simulink model "mppt"  (R2022b)
settings: Solver=ode23tb  StartTime=0.0  StopTime=0.5  RelTol=1e-3
libraries: spsSeriesRLCBranchLib x7, spsCurrentMeasurementLib x4, spsVoltageMeasurementLib x4, spsDiodeLib x2, spsIGBTDiodeLib x2, simulink x2, spsFuelCellStackLib x1, spsDCVoltageSourceLib x1, spspowerguiLib x1
settings Model: Creator=gobis  LastModifiedBy=gobis
settings SolverCC: ZeroCrossAlgorithm=Adaptive
settings DebuggingCC: MaskedZcDiagnostic=none  IgnoredZcDiagnostic=none

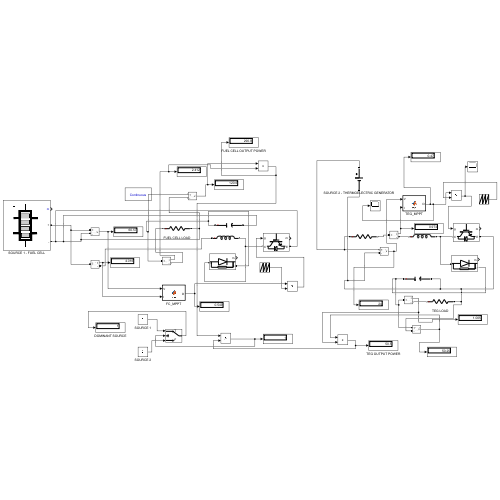
[thumbnail: Simulink's stored preview of the top-level diagram]
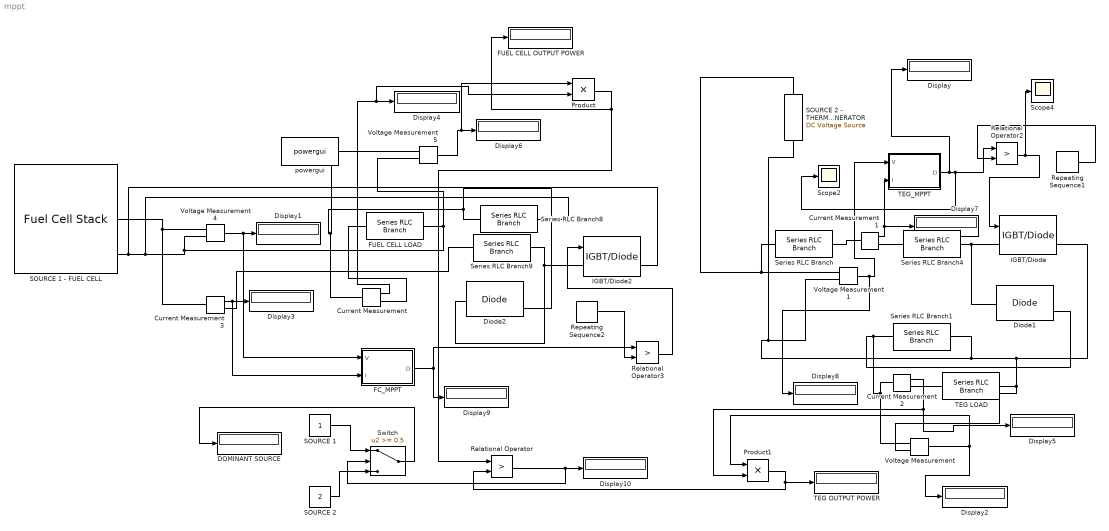
== system mppt ==
  Current Measurement{,1..3} (4 alike) : spsCurrentMeasurementLib/Current Measurement  PhasorSimulation=off  OutputType=Complex  PSBequivalent=0
  DOMINANT SOURCE : Display
  Diode1 : spsDiodeLib/Diode  Ron=0.001  Lon=0  Vf=0.8  IC=0  UseSnubber=0  Rs=500  Cs=250e-9  Measurements=on
  Diode2 : spsDiodeLib/Diode  Ron=0.001  Lon=0  Vf=0.8  IC=0  UseSnubber=0  Rs=500  Cs=250e-9  Measurements=on
  Display{,1..10} (11 alike) : Display
  FC_MPPT : MATLAB Function  TreatAsAtomicUnit=on
  FUEL CELL LOAD : spsSeriesRLCBranchLib/Series RLC Branch  LConnTagsString=__new0  RConnTagsString=__new0  BranchType=R  Resistance=50  Inductance=1e-3  SetiL0=off  InitialCurrent=0  Capacitance=1e-6  Setx0=off  InitialVoltage=0  Measurements=None
  FUEL CELL OUTPUT POWER : Display
  IGBT/Diode : spsIGBTDiodeLib/IGBT//Diode  Ron=1e-3  Rs=1e5  Cs=inf  Measurements=on
  IGBT/Diode2 : spsIGBTDiodeLib/IGBT//Diode  Ron=1e-3  Rs=1e5  Cs=inf  Measurements=on
  Product : Product
  Product1 : Product
  Relational Operator : RelationalOperator  Operator=>  OutDataTypeStr=boolean  RndMeth=Simplest  InputSameDT=off
  Relational Operator2 : RelationalOperator  Operator=>  OutDataTypeStr=boolean  RndMeth=Simplest  InputSameDT=off
  Relational Operator3 : RelationalOperator  Operator=>  OutDataTypeStr=boolean  RndMeth=Simplest  InputSameDT=off
  Repeating Sequence1 : simulink/Sources/Repeating Sequence  rep_seq_t=[0 0.0001]  rep_seq_y=[0 1]
  Repeating Sequence2 : simulink/Sources/Repeating Sequence  rep_seq_t=[0 0.0001]  rep_seq_y=[0 1]
  SOURCE 1 : Constant
  SOURCE 1 - FUEL CELL : spsFuelCellStackLib/Fuel Cell Stack  PresetModel=No (User-Defined)  FcType=0  Detailed=Detailed  Eoc=[65,63]  NomVI=[133.3,45]  EndVI=[225,37]  Nc=65  n=55  TOp=65  AirFr=300  SuppPress=[1.5,1]  Comp=[99.95,21,1]  SignX=off  SignY=off  FlowRateH2=off  FlowRateAir=off  SystemTemp=off  SystemPH2=off  SystemPAir=off  FCDyn=off  FC_tau=1  Peak_O2=80  V_Under=10
      settings: LibrarySourceBlock=sps_lib/Sources/Fuel Cell Stack
  SOURCE 2 : Constant  Value=2
  SOURCE 2 - THERMOELECTRIC GENERATOR : spsDCVoltageSourceLib/DC Voltage Source  Amplitude=24  Measurements=None
  Scope2 : Scope
  Scope4 : Scope
  Series RLC Branch : spsSeriesRLCBranchLib/Series RLC Branch  LConnTagsString=__new0  RConnTagsString=__new0  BranchType=R  Resistance=1  Inductance=1e-3  SetiL0=off  InitialCurrent=0  Capacitance=1e-6  Setx0=off  InitialVoltage=0  Measurements=None
  Series RLC Branch1 : spsSeriesRLCBranchLib/Series RLC Branch  LConnTagsString=__new0  RConnTagsString=__new0  BranchType=C  Resistance=1  Inductance=1e-3  SetiL0=off  InitialCurrent=0  Capacitance=1e-6  Setx0=off  InitialVoltage=0  Measurements=None
  Series RLC Branch4 : spsSeriesRLCBranchLib/Series RLC Branch  LConnTagsString=__new0  RConnTagsString=__new0  BranchType=L  Resistance=1  Inductance=1e-3  SetiL0=off  InitialCurrent=0  Capacitance=1e-6  Setx0=off  InitialVoltage=0  Measurements=None
  Series RLC Branch8 : spsSeriesRLCBranchLib/Series RLC Branch  LConnTagsString=__new0  RConnTagsString=__new0  BranchType=C  Resistance=1  Inductance=1e-3  SetiL0=off  InitialCurrent=0  Capacitance=470e-6  Setx0=off  InitialVoltage=0  Measurements=None
  Series RLC Branch9 : spsSeriesRLCBranchLib/Series RLC Branch  LConnTagsString=__new0  RConnTagsString=__new0  BranchType=L  Resistance=1  Inductance=1e-3  SetiL0=off  InitialCurrent=0  Capacitance=1e-6  Setx0=off  InitialVoltage=0  Measurements=None
  Switch : Switch  Threshold=0.5  SaturateOnIntegerOverflow=off  InputSameDT=off
  TEG LOAD : spsSeriesRLCBranchLib/Series RLC Branch  LConnTagsString=__new0  RConnTagsString=__new0  BranchType=R  Resistance=50  Inductance=1e-3  SetiL0=off  InitialCurrent=0  Capacitance=1e-6  Setx0=off  InitialVoltage=0  Measurements=None
  TEG OUTPUT POWER : Display
  TEG_MPPT : MATLAB Function  TreatAsAtomicUnit=on
  Voltage Measurement{,1,4..5} (4 alike) : spsVoltageMeasurementLib/Voltage Measurement  PhasorSimulation=off  OutputType=Complex  PSBequivalent=0
  powergui : spspowerguiLib/powergui  Priority=1  SimulationMode=Continuous  SampleTime=50e-6  frequency=60  Iterations=50  frequencyindice=0  Pbase=100e6  ErrMax=1e-4  UnitsV=kV  UnitsW=MW  buscounter=0  FunctionMessages=off  echomessages=off  EnableUseOfTLC=off  CurrentSourceSwitches=off  DisableSnubberDevices=off  DisableRonSwitches=off  DisableVfSwitches=off  DisplayEquations=off  AutomaticDiscreteSolvers=off  SolverType=Tustin/Backward Euler (TBE)  Interpol=off  ExternalGateDelay=off  methode=off  Ts=100  x0status=blocks  SPID=on  SwTol=0  HookPort=off  NonlinearTolerance=1e-4  nMaxIteration=100  ContinueOnMaxIteration=off  RestoreLinks=warning  ResistiveCurrentMeasurement=off  Frange=[0:2:500]  Ylog=off  Xlog=on  ShowGrid=off  save=off  variable=ZData  structure=0  ZoomFFT=off  StartTime=0.0  cycles=1  DisplayStyle=1  fundamental=60  FreqAxis=off  MaxFrequency=1000  frequencyindicesteady=1  RmsSteady=1  display=off
  wires:
  Voltage Measurement1/1 -> Display8/1, TEG_MPPT/1(V)
  Current Measurement1/1 -> Display7/1, TEG_MPPT/2(I)
  TEG_MPPT/1(D) -> Display/1, Scope2/1, Relational Operator2/1
  Repeating Sequence1/1 -> Relational Operator2/2
  Relational Operator2/1 -> Scope4/1, IGBT/Diode/1
  Current Measurement3/1 -> FC_MPPT/2(I), Display3/1
  Voltage Measurement4/1 -> FC_MPPT/1(V), Display1/1
  Voltage Measurement5/1 -> Product/1, Display6/1
  Repeating Sequence2/1 -> Relational Operator3/2
  Relational Operator3/1 -> IGBT/Diode2/1
  FC_MPPT/1(D) -> Relational Operator3/1, Display9/1
  Voltage Measurement/1 -> Display2/1, Product1/1
  Current Measurement/1 -> Product/2, Display4/1
  Current Measurement2/1 -> Product1/2, Display5/1
  Relational Operator/1 -> Switch/2, Display10/1
  Product/1 -> Relational Operator/1, FUEL CELL OUTPUT POWER/1
  Product1/1 -> TEG OUTPUT POWER/1, Relational Operator/2
  SOURCE 1/1 -> Switch/1
  SOURCE 2/1 -> Switch/3
  Switch/1 -> DOMINANT SOURCE/1
  connections:
  SOURCE 2 - THERMOELECTRIC GENERATOR/RConn1 -- Series RLC Branch/LConn1 -- Voltage Measurement1/LConn1
  IGBT/Diode/LConn1 -- Diode1/LConn1 -- Series RLC Branch4/RConn1
  Current Measurement1/RConn1 -- Series RLC Branch4/LConn1
  Current Measurement1/LConn1 -- Series RLC Branch/RConn1
  Voltage Measurement4/LConn1 -- SOURCE 1 - FUEL CELL/RConn1 -- Current Measurement3/LConn1
  Current Measurement3/RConn1 -- Series RLC Branch9/LConn1
  Series RLC Branch9/RConn1 -- Diode2/LConn1 -- IGBT/Diode2/LConn1
  IGBT/Diode/RConn1 -- Voltage Measurement/LConn2 -- TEG LOAD/RConn1 -- Series RLC Branch1/RConn1 -- Voltage Measurement1/LConn2 -- SOURCE 2 - THERMOELECTRIC GENERATOR/LConn1
  Series RLC Branch8/RConn1 -- FUEL CELL LOAD/RConn1 -- Voltage Measurement5/LConn2 -- Voltage Measurement4/LConn2 -- IGBT/Diode2/RConn1 -- SOURCE 1 - FUEL CELL/RConn2
  Diode2/RConn1 -- Current Measurement/LConn1 -- Voltage Measurement5/LConn1 -- Series RLC Branch8/LConn1
  Voltage Measurement/LConn1 -- Current Measurement2/LConn1 -- Diode1/RConn1 -- Series RLC Branch1/LConn1
  Current Measurement/RConn1 -- FUEL CELL LOAD/LConn1
  Current Measurement2/RConn1 -- TEG LOAD/LConn1

== matlab function mppt/FC_MPPT ==
  settings: updateMethod=DISCRETE
  data: V input; D output; I input
function D = fcn(V,I)

persistent Dprev Pprev dir

if isempty(Dprev)
    Dprev = 0.53;
    Pprev = 0;
    dir = 1;
end

P = V*I;

if P > Pprev
    D = Dprev + dir*0.001;
else
    dir = -dir;
    D = Dprev + dir*0.001;
end

D = min(max(D,0.3),0.7);

Pprev = P;
Dprev = D;

end

== matlab function mppt/TEG_MPPT ==
  settings: updateMethod=DISCRETE
  data: V input; D output; I input
function D = fcn(V,I)

persistent Dprev Pprev dir

if isempty(Dprev)
    Dprev = 0.5;
    Pprev = 0;
    dir = 1;
end

P = V*I;

if P > Pprev
    D = Dprev + dir*0.01;
else
    dir = -dir;
    D = Dprev + dir*0.01;
end

D = min(max(D,0.1),0.9);

Pprev = P;
Dprev = D;

end
